simulink model "sim1"  (R2015b)
settings: Solver=VariableStepAuto  StartTime=0.0  StopTime=20  RelTol=1e-3
values from neighbouring files (symbols this model uses):
  A2 = [0 1 0 ... (first row only)    [tp1.m]
  B2 = [0 ... (first row only)    [tp1.m]
  K2 = place(A2,B2,[lmb(1) lmb(2) 0])    [tp1.m]
settings Model: Creator=max.Sonzogni  LastModifiedBy=max.sonzogni

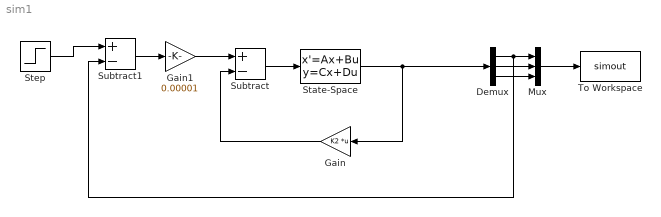
== system sim1 ==
  Demux : Demux  Outputs=3
  Gain : Gain  Gain=K2  Multiplication=Matrix(K*u)
  Gain1 : Gain  Gain=0.00001
  Mux : Mux  Inputs=3
  State-Space : StateSpace  A=A2  B=B2  C=eye(3)  D=zeros(3,1)  X0=0
  Step : Step  Time=0  SampleTime=0
  Subtract : Sum  Inputs=+-
  Subtract1 : Sum  Inputs=+-
  To Workspace : ToWorkspace  VariableName=simout  SampleTime=-1
  wires:
  State-Space/1 -> Demux/1, Gain/1
  Subtract/1 -> State-Space/1
  Gain/1 -> Subtract/2
  Demux/2 -> Mux/2
  Step/1 -> Subtract1/1
  Mux/1 -> To Workspace/1
  Demux/3 -> Mux/3
  Demux/1 -> Subtract1/2, Mux/1
  Gain1/1 -> Subtract/1
  Subtract1/1 -> Gain1/1
